simulink model "gm_buz_del"  (R2018b)
settings: Solver=FixedStepDiscrete  StartTime=0.0  StopTime=10.0  RelTol=1e-3
libraries: dspvision x2
settings Model: Creator=Mohaddeseh  LastModifiedBy=Mohaddeseh
settings DataIOCC: LimitDataPoints=on  SaveOutput=off  SaveTime=off
settings OptimizationCC: BlockReduction=off  ConditionallyExecuteInputs=off  DefaultParameterBehavior=Inlined  LifeSpan=inf
settings DebuggingCC: AlgebraicLoopMsg=error  InheritedTsInSrcMsg=none  SingleTaskRateTransMsg=error  AllowSymbolicDim=off  StrictBusMsg=ErrorOnBusTreatedAsVector  SFUnexpectedBacktrackingDiag=warning  SFNoUnconditionalDefaultTransitionDiag=warning  SFExecutionAtInitializationDiag=none
settings HardwareCC: ProdBitPerPointer=32  ProdBitPerSizeT=32  ProdBitPerPtrDiffT=32  ProdLargestAtomicFloat=None  ProdIntDivRoundTo=Undefined  ProdEndianess=Unspecified  ProdWordSize=32  ProdHWDeviceType=ASIC/FPGA->ASIC/FPGA  ProdEqTarget=off
settings SFSimCC: SimUseLocalCustomCode=off
settings RTWCC: RTWUseLocalCustomCode=off
settings CodeAppCC: StateflowObjectComments=on
settings GRTTargetCC: TargetLangStandard=C89/C90 (ANSI)  GeneratePreprocessorConditionals=Disable all
settings ConfigComp: CovScope=ReferencedModels  CovMetricSettings=dw  CovHtmlReporting=on  CovSaveCumulativeToWorkspaceVar=on  CovSaveSingleToWorkspaceVar=on  CovExternalEMLEnable=off  CovSFcnEnable=off

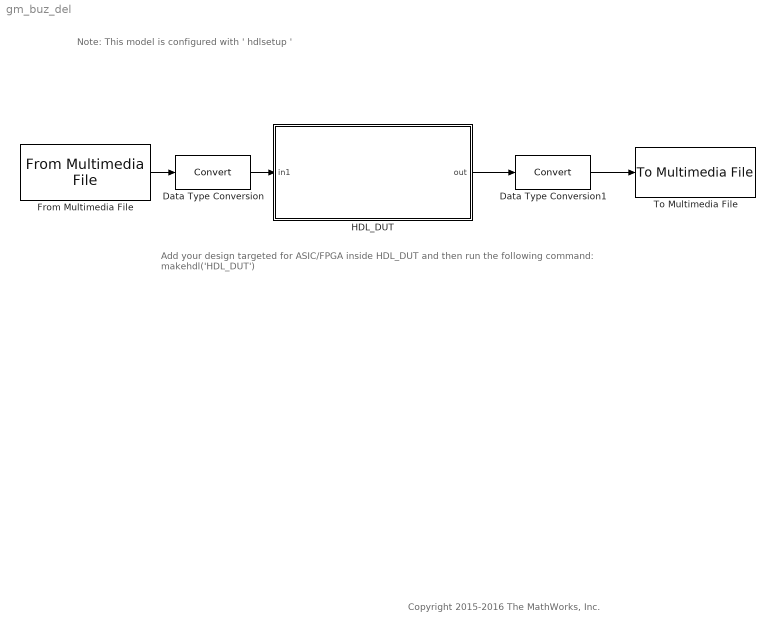
== system gm_buz_del ==
  note: Copyright 2015-2016 The MathWorks, Inc.
  note: Add your design targeted for ASIC/FPGA inside HDL_DUT and then run the following command:
      | makehdl('HDL_DUT')
  note: Note: This model is configured with ' hdlsetup '
  Data Type Conversion : DataTypeConversion  RndMeth=Nearest
  Data Type Conversion1 : DataTypeConversion  RndMeth=Nearest
  From Multimedia File : dspvision/From Multimedia File  inputFilename=F:\fpga lab\exp1\hum.wav  loop=on  numPlays=1  outputStreams=Audio only  videoDataType=single  audioDataType=double  inheritSampleTime=on  userDefinedSampleTime=1/30  noAudioOutput=off  isIntensityVideo=off  fourcc=RGB  colorVideoFormat=Separate color signals  outputEOF=off  dataOrg=Column-major  audioFrameSize=1  computeAudioFrameSize=off  outSamplingMode=Sample based
      settings: SourceProductBaseCode=VP
  HDL_DUT : Subsystem
  To Multimedia File : dspvision/To Multimedia File  outputFilename=F:\fpga lab\exp1\filtered_audio.wav  streamSelection=Audio only  videoCompressor=None (uncompressed)  audioCompressor=None (uncompressed)  imagePorts=Separate color signals  fileType=WAV  audioDatatype=16-bit integer  fourcc=RGB  videoQuality=75  mj2000CompFactor=10
      settings: SourceProductName=Computer Vision System Toolbox  SourceProductBaseCode=VP
  wires:
  Data Type Conversion1/1 -> To Multimedia File/1
  HDL_DUT/1(out) -> Data Type Conversion1/1
  From Multimedia File/1 -> Data Type Conversion/1
  Data Type Conversion/1 -> HDL_DUT/1(in1)

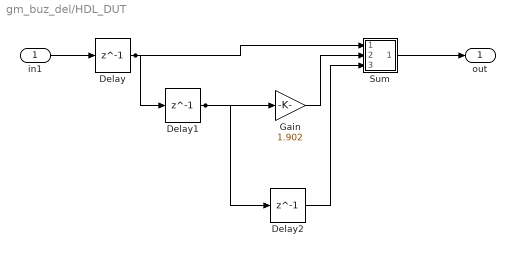
== system gm_buz_del/HDL_DUT ==
  in1 : Inport  OutDataTypeStr=fixdt(1, 16, 15)  PortDimensions=1  SampleTime=0.000125
  Delay : Delay  DelayLength=1  InitialCondition=0
  Delay1 : Delay  DelayLength=1  InitialCondition=0
  Delay2 : Delay  DelayLength=1  InitialCondition=0
  Gain : Gain  Gain=1.902  OutDataTypeStr=fixdt(1,16,14)  RndMeth=Nearest
  Sum : Subsystem
  out : Outport
  wires:
  in1/1 -> Delay/1
  Delay/1 -> Sum/1(In1), Delay1/1
  Delay1/1 -> Gain/1, Delay2/1
  Delay2/1 -> Sum/3(In3)
  Gain/1 -> Sum/2(In2)
  Sum/1(Out1) -> out/1

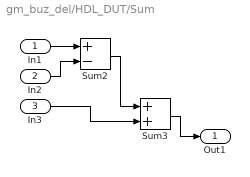
== system gm_buz_del/HDL_DUT/Sum ==
  In1 : Inport  OutDataTypeStr=fixdt('sfix16_En15')
  In2 : Inport  Port=2  OutDataTypeStr=fixdt('sfix16_En14')
  In3 : Inport  Port=3  OutDataTypeStr=fixdt('sfix16_En15')
  Sum2 : Sum  Inputs=+-  AccumDataTypeStr=fixdt(1,18,15)  OutDataTypeStr=fixdt(1,18,15)  RndMeth=Nearest
  Sum3 : Sum  AccumDataTypeStr=fixdt(1,18,15)  OutDataTypeStr=fixdt(1,18,15)  RndMeth=Nearest
  Out1 : Outport
  wires:
  In1/1 -> Sum2/1
  In2/1 -> Sum2/2
  Sum2/1 -> Sum3/1
  In3/1 -> Sum3/2
  Sum3/1 -> Out1/1
